simulink model "MIMO_FLOATING_POINT"  (R2023b)
settings: Solver=VariableStepAuto  StartTime=0.0  StopTime=1000  RelTol=1e-3
libraries: dspsigops x80, commchan3 x4, commdigbbndpm3 x2, commfilt2 x2, commsink2 x1, simulink x1, commrandsrc3 x1
(part 3 of 3)

== system MIMO_FLOATING_POINT/Transceiver5/Interpolation /E1(Z) ==
  Input1 : Inport
  10-12 : Gain  Gain=0.3078
  2-20 : Gain  Gain=0.0011
  4-18 : Gain  Gain=-0.0072
  6-16 : Gain  Gain=0.0263
  8-14 : Gain  Gain=-0.078
  Add{7..10,12..16} (9 alike) : Sum
  Delay{21,23,25,27,29,31,33,35,37} (9 alike) : Delay  DelayLength=1
  Output : Outport
  wires:
  8-14/1 -> Add13/1, Add9/1
  Delay29/1 -> Add12/2  "x[n-11]"
  Add14/1 -> Delay35/1
  Input1/1 -> 2-20/1, 4-18/1, 6-16/1, 8-14/1, 10-12/1
  Add8/1 -> Delay25/1
  4-18/1 -> Add15/1, Add7/1
  Delay33/1 -> Add14/2  "x[n-15]"
  Add12/1 -> Delay31/1
  10-12/1 -> Add10/1, Add12/1
  Add9/1 -> Delay27/1
  Add16/1 -> Output/1
  Delay37/1 -> Add16/2  "x[n-19]"
  6-16/1 -> Add14/1, Add8/1
  Delay25/1 -> Add9/2  "x[n-7]"
  Add7/1 -> Delay23/1
  Add15/1 -> Delay37/1
  Delay23/1 -> Add8/2  "x[n-5]"
  Delay27/1 -> Add10/2  "x[n-9]"
  Delay31/1 -> Add13/2  "x[n-13]"
  Delay35/1 -> Add15/2  "x[n-17]"
  Delay21/1 -> Add7/2  "x[n-3]"
  2-20/1 -> Delay21/1, Add16/1
  Add13/1 -> Delay33/1
  Add10/1 -> Delay29/1

== system MIMO_FLOATING_POINT/Transceiver5/Interpolation /E2 ==
  In1 : Inport
  Delay3 : Delay  DelayLength=1
  Delay4 : Delay  DelayLength=1
  Delay5 : Delay  DelayLength=1
  Gain : Gain  Gain=10
  Gain1 : Gain  Gain=246
  Sum : Sum
  Sum1 : Sum
  Sum2 : Sum
  Out1 : Outport
  wires:
  In1/1 -> Gain1/1, Gain/1
  Sum1/1 -> Delay5/1
  Sum/1 -> Delay4/1
  Gain1/1 -> Sum1/1, Sum/1
  Delay3/1 -> Sum/2
  Delay4/1 -> Sum1/2
  Gain/1 -> Sum2/1, Delay3/1
  Delay5/1 -> Sum2/2
  Sum2/1 -> Out1/1

== system MIMO_FLOATING_POINT/Transceiver5/Interpolation /E3 ==
  In1 : Inport
  Delay3 : Delay  DelayLength=1
  Delay4 : Delay  DelayLength=1
  Delay5 : Delay  DelayLength=1
  Gain : Gain  Gain=4
  Gain1 : Gain  Gain=204
  Gain2 : Gain  Gain=284
  Gain3 : Gain  Gain=20
  Sum : Sum
  Sum1 : Sum
  Sum2 : Sum
  Out1 : Outport
  wires:
  In1/1 -> Gain2/1, Gain3/1, Gain1/1, Gain/1
  Sum1/1 -> Delay5/1
  Sum/1 -> Delay4/1
  Gain1/1 -> Sum/1
  Delay3/1 -> Sum/2
  Delay4/1 -> Sum1/2
  Gain3/1 -> Sum2/1
  Delay5/1 -> Sum2/2
  Gain/1 -> Delay3/1
  Sum2/1 -> Out1/1
  Gain2/1 -> Sum1/1

== system MIMO_FLOATING_POINT/Transceiver5/Interpolation /E4 ==
  In1 : Inport
  Delay3 : Delay  DelayLength=1
  Delay4 : Delay  DelayLength=1
  Delay5 : Delay  DelayLength=1
  Gain : Gain
  Gain1 : Gain  Gain=161
  Gain2 : Gain  Gain=315
  Gain3 : Gain  Gain=35
  Sum : Sum
  Sum1 : Sum
  Sum2 : Sum
  Out1 : Outport
  wires:
  In1/1 -> Gain2/1, Gain3/1, Gain1/1, Gain/1
  Sum1/1 -> Delay5/1
  Sum/1 -> Delay4/1
  Gain1/1 -> Sum/1
  Delay3/1 -> Sum/2
  Delay4/1 -> Sum1/2
  Gain3/1 -> Sum2/1
  Delay5/1 -> Sum2/2
  Gain/1 -> Delay3/1
  Sum2/1 -> Out1/1
  Gain2/1 -> Sum1/1

== system MIMO_FLOATING_POINT/Transceiver5/Interpolation /E5 ==
  In1 : Inport
  Delay6 : Delay  DelayLength=1
  Delay7 : Delay  DelayLength=1
  Gain4 : Gain  Gain=120
  Gain5 : Gain  Gain=336
  Gain6 : Gain  Gain=56
  Sum4 : Sum
  Sum5 : Sum
  Out1 : Outport
  wires:
  Gain4/1 -> Delay6/1
  In1/1 -> Gain6/1, Gain5/1, Gain4/1
  Sum5/1 -> Out1/1
  Sum4/1 -> Delay7/1
  Delay7/1 -> Sum5/2
  Gain6/1 -> Sum5/1
  Gain5/1 -> Sum4/1
  Delay6/1 -> Sum4/2

== system MIMO_FLOATING_POINT/Transceiver5/Interpolation /E6 ==
  In1 : Inport
  Delay6 : Delay  DelayLength=1
  Delay7 : Delay  DelayLength=1
  Gain4 : Gain  Gain=84
  Gain5 : Gain  Gain=344
  Sum4 : Sum
  Sum5 : Sum
  Out1 : Outport
  wires:
  In1/1 -> Gain5/1, Gain4/1
  Sum5/1 -> Out1/1
  Sum4/1 -> Delay7/1
  Delay7/1 -> Sum5/2
  Gain4/1 -> Sum5/1, Delay6/1
  Gain5/1 -> Sum4/1
  Delay6/1 -> Sum4/2

== system MIMO_FLOATING_POINT/Transceiver5/Interpolation /E7 ==
  In1 : Inport
  Delay6 : Delay  DelayLength=1
  Delay7 : Delay  DelayLength=1
  Gain4 : Gain  Gain=56
  Gain5 : Gain  Gain=336
  Gain6 : Gain  Gain=120
  Sum4 : Sum
  Sum5 : Sum
  Out1 : Outport
  wires:
  Gain4/1 -> Delay6/1
  In1/1 -> Gain6/1, Gain5/1, Gain4/1
  Sum5/1 -> Out1/1
  Sum4/1 -> Delay7/1
  Delay7/1 -> Sum5/2
  Gain6/1 -> Sum5/1
  Gain5/1 -> Sum4/1
  Delay6/1 -> Sum4/2

== system MIMO_FLOATING_POINT/Transceiver5/Interpolation 1/E0 ==
  In1 : Inport
  Delay3 : Delay  DelayLength=1
  Delay4 : Delay  DelayLength=1
  Delay5 : Delay  DelayLength=1
  Gain : Gain  Gain=35
  Gain1 : Gain  Gain=315
  Gain2 : Gain  Gain=161
  Gain3 : Gain
  Sum : Sum
  Sum1 : Sum
  Sum2 : Sum
  Out1 : Outport
  wires:
  In1/1 -> Gain2/1, Gain3/1, Gain1/1, Gain/1
  Sum1/1 -> Delay5/1
  Sum/1 -> Delay4/1
  Gain1/1 -> Sum/1
  Delay3/1 -> Sum/2
  Delay4/1 -> Sum1/2
  Gain3/1 -> Sum2/1
  Delay5/1 -> Sum2/2
  Gain/1 -> Delay3/1
  Sum2/1 -> Out1/1
  Gain2/1 -> Sum1/1

== system MIMO_FLOATING_POINT/Transceiver5/Interpolation 1/E0(Z) ==
  Input : Inport
  Delay : Delay  DelayLength=5
  Gain : Gain  Gain=0.5
  Out1 : Outport
  wires:
  Input/1 -> Gain/1
  Delay/1 -> Out1/1
  Gain/1 -> Delay/1

== system MIMO_FLOATING_POINT/Transceiver5/Interpolation 1/E1 ==
  In1 : Inport
  Delay3 : Delay  DelayLength=1
  Delay4 : Delay  DelayLength=1
  Delay5 : Delay  DelayLength=1
  Gain : Gain  Gain=20
  Gain1 : Gain  Gain=284
  Gain2 : Gain  Gain=204
  Gain3 : Gain  Gain=4
  Sum : Sum
  Sum1 : Sum
  Sum2 : Sum
  Out1 : Outport
  wires:
  In1/1 -> Gain2/1, Gain3/1, Gain1/1, Gain/1
  Sum1/1 -> Delay5/1
  Sum/1 -> Delay4/1
  Gain1/1 -> Sum/1
  Delay3/1 -> Sum/2
  Delay4/1 -> Sum1/2
  Gain3/1 -> Sum2/1
  Delay5/1 -> Sum2/2
  Gain/1 -> Delay3/1
  Sum2/1 -> Out1/1
  Gain2/1 -> Sum1/1

== system MIMO_FLOATING_POINT/Transceiver5/Interpolation 1/E1(Z) ==
  Input1 : Inport
  10-12 : Gain  Gain=0.3078
  2-20 : Gain  Gain=0.0011
  4-18 : Gain  Gain=-0.0072
  6-16 : Gain  Gain=0.0263
  8-14 : Gain  Gain=-0.078
  Add{7..10,12..16} (9 alike) : Sum
  Delay{21,23,25,27,29,31,33,35,37} (9 alike) : Delay  DelayLength=1
  Output : Outport
  wires:
  8-14/1 -> Add13/1, Add9/1
  Delay29/1 -> Add12/2  "x[n-11]"
  Add14/1 -> Delay35/1
  Input1/1 -> 2-20/1, 4-18/1, 6-16/1, 8-14/1, 10-12/1
  Add8/1 -> Delay25/1
  4-18/1 -> Add15/1, Add7/1
  Delay33/1 -> Add14/2  "x[n-15]"
  Add12/1 -> Delay31/1
  10-12/1 -> Add10/1, Add12/1
  Add9/1 -> Delay27/1
  Add16/1 -> Output/1
  Delay37/1 -> Add16/2  "x[n-19]"
  6-16/1 -> Add14/1, Add8/1
  Delay25/1 -> Add9/2  "x[n-7]"
  Add7/1 -> Delay23/1
  Add15/1 -> Delay37/1
  Delay23/1 -> Add8/2  "x[n-5]"
  Delay27/1 -> Add10/2  "x[n-9]"
  Delay31/1 -> Add13/2  "x[n-13]"
  Delay35/1 -> Add15/2  "x[n-17]"
  Delay21/1 -> Add7/2  "x[n-3]"
  2-20/1 -> Delay21/1, Add16/1
  Add13/1 -> Delay33/1
  Add10/1 -> Delay29/1

== system MIMO_FLOATING_POINT/Transceiver5/Interpolation 1/E2 ==
  In1 : Inport
  Delay3 : Delay  DelayLength=1
  Delay4 : Delay  DelayLength=1
  Delay5 : Delay  DelayLength=1
  Gain : Gain  Gain=10
  Gain1 : Gain  Gain=246
  Sum : Sum
  Sum1 : Sum
  Sum2 : Sum
  Out1 : Outport
  wires:
  In1/1 -> Gain1/1, Gain/1
  Sum1/1 -> Delay5/1
  Sum/1 -> Delay4/1
  Gain1/1 -> Sum1/1, Sum/1
  Delay3/1 -> Sum/2
  Delay4/1 -> Sum1/2
  Gain/1 -> Sum2/1, Delay3/1
  Delay5/1 -> Sum2/2
  Sum2/1 -> Out1/1

== system MIMO_FLOATING_POINT/Transceiver5/Interpolation 1/E3 ==
  In1 : Inport
  Delay3 : Delay  DelayLength=1
  Delay4 : Delay  DelayLength=1
  Delay5 : Delay  DelayLength=1
  Gain : Gain  Gain=4
  Gain1 : Gain  Gain=204
  Gain2 : Gain  Gain=284
  Gain3 : Gain  Gain=20
  Sum : Sum
  Sum1 : Sum
  Sum2 : Sum
  Out1 : Outport
  wires:
  In1/1 -> Gain2/1, Gain3/1, Gain1/1, Gain/1
  Sum1/1 -> Delay5/1
  Sum/1 -> Delay4/1
  Gain1/1 -> Sum/1
  Delay3/1 -> Sum/2
  Delay4/1 -> Sum1/2
  Gain3/1 -> Sum2/1
  Delay5/1 -> Sum2/2
  Gain/1 -> Delay3/1
  Sum2/1 -> Out1/1
  Gain2/1 -> Sum1/1

== system MIMO_FLOATING_POINT/Transceiver5/Interpolation 1/E4 ==
  In1 : Inport
  Delay3 : Delay  DelayLength=1
  Delay4 : Delay  DelayLength=1
  Delay5 : Delay  DelayLength=1
  Gain : Gain
  Gain1 : Gain  Gain=161
  Gain2 : Gain  Gain=315
  Gain3 : Gain  Gain=35
  Sum : Sum
  Sum1 : Sum
  Sum2 : Sum
  Out1 : Outport
  wires:
  In1/1 -> Gain2/1, Gain3/1, Gain1/1, Gain/1
  Sum1/1 -> Delay5/1
  Sum/1 -> Delay4/1
  Gain1/1 -> Sum/1
  Delay3/1 -> Sum/2
  Delay4/1 -> Sum1/2
  Gain3/1 -> Sum2/1
  Delay5/1 -> Sum2/2
  Gain/1 -> Delay3/1
  Sum2/1 -> Out1/1
  Gain2/1 -> Sum1/1

== system MIMO_FLOATING_POINT/Transceiver5/Interpolation 1/E5 ==
  In1 : Inport
  Delay6 : Delay  DelayLength=1
  Delay7 : Delay  DelayLength=1
  Gain4 : Gain  Gain=120
  Gain5 : Gain  Gain=336
  Gain6 : Gain  Gain=56
  Sum4 : Sum
  Sum5 : Sum
  Out1 : Outport
  wires:
  Gain4/1 -> Delay6/1
  In1/1 -> Gain6/1, Gain5/1, Gain4/1
  Sum5/1 -> Out1/1
  Sum4/1 -> Delay7/1
  Delay7/1 -> Sum5/2
  Gain6/1 -> Sum5/1
  Gain5/1 -> Sum4/1
  Delay6/1 -> Sum4/2

== system MIMO_FLOATING_POINT/Transceiver5/Interpolation 1/E6 ==
  In1 : Inport
  Delay6 : Delay  DelayLength=1
  Delay7 : Delay  DelayLength=1
  Gain4 : Gain  Gain=84
  Gain5 : Gain  Gain=344
  Sum4 : Sum
  Sum5 : Sum
  Out1 : Outport
  wires:
  In1/1 -> Gain5/1, Gain4/1
  Sum5/1 -> Out1/1
  Sum4/1 -> Delay7/1
  Delay7/1 -> Sum5/2
  Gain4/1 -> Sum5/1, Delay6/1
  Gain5/1 -> Sum4/1
  Delay6/1 -> Sum4/2

== system MIMO_FLOATING_POINT/Transceiver5/Interpolation 1/E7 ==
  In1 : Inport
  Delay6 : Delay  DelayLength=1
  Delay7 : Delay  DelayLength=1
  Gain4 : Gain  Gain=56
  Gain5 : Gain  Gain=336
  Gain6 : Gain  Gain=120
  Sum4 : Sum
  Sum5 : Sum
  Out1 : Outport
  wires:
  Gain4/1 -> Delay6/1
  In1/1 -> Gain6/1, Gain5/1, Gain4/1
  Sum5/1 -> Out1/1
  Sum4/1 -> Delay7/1
  Delay7/1 -> Sum5/2
  Gain6/1 -> Sum5/1
  Gain5/1 -> Sum4/1
  Delay6/1 -> Sum4/2

== system MIMO_FLOATING_POINT/Transceiver6/ADC 1/SigmaDelta ADC ==
  note: c1
  In : Inport
  Discrete Transfer Fcn : DiscreteTransferFcn  Denominator=[1 -1]
  Discrete Transfer Fcn1 : DiscreteTransferFcn  Numerator=[1 0]  Denominator=[1 -1]
  Discrete Transfer Fcn2 : DiscreteTransferFcn  Denominator=[1 -1]
  Discrete Transfer Fcn3 : DiscreteTransferFcn  Numerator=[1 0]  Denominator=[1 -1]
  Discrete Transfer Fcn4 : DiscreteTransferFcn  Denominator=[1 -1]
  Discrete Transfer Fcn5 : DiscreteTransferFcn  Numerator=[1 0]  Denominator=[1 -1]
  Sign : Signum
  Sum : Sum  Inputs=-++  InputSameDT=on  SaturateOnIntegerOverflow=on  OutDataTypeStr=Inherit: Same as first input
  Sum1 : Sum  Inputs=-+  InputSameDT=on  SaturateOnIntegerOverflow=on  OutDataTypeStr=Inherit: Same as first input
  Sum3 : Sum  Inputs=-+  InputSameDT=on  SaturateOnIntegerOverflow=on  OutDataTypeStr=Inherit: Same as first input
  Sum4 : Sum  Inputs=++++++  InputSameDT=on  SaturateOnIntegerOverflow=on  OutDataTypeStr=Inherit: Same as first input
  a : Gain  Gain=-1  SaturateOnIntegerOverflow=on  OutDataTypeStr=Inherit: Same as input  ParamDataTypeStr=Inherit: Same as input
  a1 : Gain  Gain=0.556869897897495  SaturateOnIntegerOverflow=on  OutDataTypeStr=Inherit: Same as input  ParamDataTypeStr=Inherit: Same as input
  a2 : Gain  Gain=-0.556869897925717  SaturateOnIntegerOverflow=on  OutDataTypeStr=Inherit: Same as input  ParamDataTypeStr=Inherit: Same as input
  a3 : Gain  Gain=5.57074843011795e-10  SaturateOnIntegerOverflow=on  OutDataTypeStr=Inherit: Same as input  ParamDataTypeStr=Inherit: Same as input
  a4 : Gain  Gain=-0.239860502762260  SaturateOnIntegerOverflow=on  OutDataTypeStr=Inherit: Same as input  ParamDataTypeStr=Inherit: Same as input
  a5 : Gain  Gain=-0.0411685762497780  SaturateOnIntegerOverflow=on  OutDataTypeStr=Inherit: Same as input  ParamDataTypeStr=Inherit: Same as input
  a6 : Gain  Gain=0.0229325751731016  SaturateOnIntegerOverflow=on  OutDataTypeStr=Inherit: Same as input  ParamDataTypeStr=Inherit: Same as input
  gc1 : Gain  Gain=2.00000000000000  SaturateOnIntegerOverflow=on  OutDataTypeStr=Inherit: Same as input  ParamDataTypeStr=Inherit: Same as input
  gc2 : Gain  Gain=2.07602752770857  SaturateOnIntegerOverflow=on  OutDataTypeStr=Inherit: Same as input  ParamDataTypeStr=Inherit: Same as input
  gc3 : Gain  Gain=1.92397247229143  SaturateOnIntegerOverflow=on  OutDataTypeStr=Inherit: Same as input  ParamDataTypeStr=Inherit: Same as input
  Out : Outport
  wires:
  gc1/1 -> Sum/1
  a5/1 -> Sum4/2
  Discrete Transfer Fcn2/1 -> Discrete Transfer Fcn3/1, a3/1
  Sum4/1 -> Sign/1
  Sum1/1 -> Discrete Transfer Fcn2/1
  Sum/1 -> Discrete Transfer Fcn/1
  a1/1 -> Sum4/6
  gc2/1 -> Sum1/1
  a/1 -> Sum/3
  Discrete Transfer Fcn3/1 -> a4/1, Sum3/2, gc2/1
  Discrete Transfer Fcn5/1 -> a6/1, gc3/1
  Discrete Transfer Fcn1/1 -> a2/1, gc1/1, Sum1/2
  In/1 -> Sum/2
  Sign/1 -> Out/1, a/1
  gc3/1 -> Sum3/1
  a3/1 -> Sum4/4
  a4/1 -> Sum4/3
  a2/1 -> Sum4/5
  Discrete Transfer Fcn/1 -> Discrete Transfer Fcn1/1, a1/1
  Sum3/1 -> Discrete Transfer Fcn4/1
  Discrete Transfer Fcn4/1 -> Discrete Transfer Fcn5/1, a5/1
  a6/1 -> Sum4/1

== system MIMO_FLOATING_POINT/Transceiver6/Interpolation /E0 ==
  In1 : Inport
  Delay3 : Delay  DelayLength=1
  Delay4 : Delay  DelayLength=1
  Delay5 : Delay  DelayLength=1
  Gain : Gain  Gain=35
  Gain1 : Gain  Gain=315
  Gain2 : Gain  Gain=161
  Gain3 : Gain
  Sum : Sum
  Sum1 : Sum
  Sum2 : Sum
  Out1 : Outport
  wires:
  In1/1 -> Gain2/1, Gain3/1, Gain1/1, Gain/1
  Sum1/1 -> Delay5/1
  Sum/1 -> Delay4/1
  Gain1/1 -> Sum/1
  Delay3/1 -> Sum/2
  Delay4/1 -> Sum1/2
  Gain3/1 -> Sum2/1
  Delay5/1 -> Sum2/2
  Gain/1 -> Delay3/1
  Sum2/1 -> Out1/1
  Gain2/1 -> Sum1/1

== system MIMO_FLOATING_POINT/Transceiver6/Interpolation /E0(Z) ==
  Input : Inport
  Delay : Delay  DelayLength=5
  Gain : Gain  Gain=0.5
  Out1 : Outport
  wires:
  Input/1 -> Gain/1
  Delay/1 -> Out1/1
  Gain/1 -> Delay/1

== system MIMO_FLOATING_POINT/Transceiver6/Interpolation /E1 ==
  In1 : Inport
  Delay3 : Delay  DelayLength=1
  Delay4 : Delay  DelayLength=1
  Delay5 : Delay  DelayLength=1
  Gain : Gain  Gain=20
  Gain1 : Gain  Gain=284
  Gain2 : Gain  Gain=204
  Gain3 : Gain  Gain=4
  Sum : Sum
  Sum1 : Sum
  Sum2 : Sum
  Out1 : Outport
  wires:
  In1/1 -> Gain2/1, Gain3/1, Gain1/1, Gain/1
  Sum1/1 -> Delay5/1
  Sum/1 -> Delay4/1
  Gain1/1 -> Sum/1
  Delay3/1 -> Sum/2
  Delay4/1 -> Sum1/2
  Gain3/1 -> Sum2/1
  Delay5/1 -> Sum2/2
  Gain/1 -> Delay3/1
  Sum2/1 -> Out1/1
  Gain2/1 -> Sum1/1

== system MIMO_FLOATING_POINT/Transceiver6/Interpolation /E1(Z) ==
  Input1 : Inport
  10-12 : Gain  Gain=0.3078
  2-20 : Gain  Gain=0.0011
  4-18 : Gain  Gain=-0.0072
  6-16 : Gain  Gain=0.0263
  8-14 : Gain  Gain=-0.078
  Add{7..10,12..16} (9 alike) : Sum
  Delay{21,23,25,27,29,31,33,35,37} (9 alike) : Delay  DelayLength=1
  Output : Outport
  wires:
  8-14/1 -> Add13/1, Add9/1
  Delay29/1 -> Add12/2  "x[n-11]"
  Add14/1 -> Delay35/1
  Input1/1 -> 2-20/1, 4-18/1, 6-16/1, 8-14/1, 10-12/1
  Add8/1 -> Delay25/1
  4-18/1 -> Add15/1, Add7/1
  Delay33/1 -> Add14/2  "x[n-15]"
  Add12/1 -> Delay31/1
  10-12/1 -> Add10/1, Add12/1
  Add9/1 -> Delay27/1
  Add16/1 -> Output/1
  Delay37/1 -> Add16/2  "x[n-19]"
  6-16/1 -> Add14/1, Add8/1
  Delay25/1 -> Add9/2  "x[n-7]"
  Add7/1 -> Delay23/1
  Add15/1 -> Delay37/1
  Delay23/1 -> Add8/2  "x[n-5]"
  Delay27/1 -> Add10/2  "x[n-9]"
  Delay31/1 -> Add13/2  "x[n-13]"
  Delay35/1 -> Add15/2  "x[n-17]"
  Delay21/1 -> Add7/2  "x[n-3]"
  2-20/1 -> Delay21/1, Add16/1
  Add13/1 -> Delay33/1
  Add10/1 -> Delay29/1

== system MIMO_FLOATING_POINT/Transceiver6/Interpolation /E2 ==
  In1 : Inport
  Delay3 : Delay  DelayLength=1
  Delay4 : Delay  DelayLength=1
  Delay5 : Delay  DelayLength=1
  Gain : Gain  Gain=10
  Gain1 : Gain  Gain=246
  Sum : Sum
  Sum1 : Sum
  Sum2 : Sum
  Out1 : Outport
  wires:
  In1/1 -> Gain1/1, Gain/1
  Sum1/1 -> Delay5/1
  Sum/1 -> Delay4/1
  Gain1/1 -> Sum1/1, Sum/1
  Delay3/1 -> Sum/2
  Delay4/1 -> Sum1/2
  Gain/1 -> Sum2/1, Delay3/1
  Delay5/1 -> Sum2/2
  Sum2/1 -> Out1/1

== system MIMO_FLOATING_POINT/Transceiver6/Interpolation /E3 ==
  In1 : Inport
  Delay3 : Delay  DelayLength=1
  Delay4 : Delay  DelayLength=1
  Delay5 : Delay  DelayLength=1
  Gain : Gain  Gain=4
  Gain1 : Gain  Gain=204
  Gain2 : Gain  Gain=284
  Gain3 : Gain  Gain=20
  Sum : Sum
  Sum1 : Sum
  Sum2 : Sum
  Out1 : Outport
  wires:
  In1/1 -> Gain2/1, Gain3/1, Gain1/1, Gain/1
  Sum1/1 -> Delay5/1
  Sum/1 -> Delay4/1
  Gain1/1 -> Sum/1
  Delay3/1 -> Sum/2
  Delay4/1 -> Sum1/2
  Gain3/1 -> Sum2/1
  Delay5/1 -> Sum2/2
  Gain/1 -> Delay3/1
  Sum2/1 -> Out1/1
  Gain2/1 -> Sum1/1

== system MIMO_FLOATING_POINT/Transceiver6/Interpolation /E4 ==
  In1 : Inport
  Delay3 : Delay  DelayLength=1
  Delay4 : Delay  DelayLength=1
  Delay5 : Delay  DelayLength=1
  Gain : Gain
  Gain1 : Gain  Gain=161
  Gain2 : Gain  Gain=315
  Gain3 : Gain  Gain=35
  Sum : Sum
  Sum1 : Sum
  Sum2 : Sum
  Out1 : Outport
  wires:
  In1/1 -> Gain2/1, Gain3/1, Gain1/1, Gain/1
  Sum1/1 -> Delay5/1
  Sum/1 -> Delay4/1
  Gain1/1 -> Sum/1
  Delay3/1 -> Sum/2
  Delay4/1 -> Sum1/2
  Gain3/1 -> Sum2/1
  Delay5/1 -> Sum2/2
  Gain/1 -> Delay3/1
  Sum2/1 -> Out1/1
  Gain2/1 -> Sum1/1

== system MIMO_FLOATING_POINT/Transceiver6/Interpolation /E5 ==
  In1 : Inport
  Delay6 : Delay  DelayLength=1
  Delay7 : Delay  DelayLength=1
  Gain4 : Gain  Gain=120
  Gain5 : Gain  Gain=336
  Gain6 : Gain  Gain=56
  Sum4 : Sum
  Sum5 : Sum
  Out1 : Outport
  wires:
  Gain4/1 -> Delay6/1
  In1/1 -> Gain6/1, Gain5/1, Gain4/1
  Sum5/1 -> Out1/1
  Sum4/1 -> Delay7/1
  Delay7/1 -> Sum5/2
  Gain6/1 -> Sum5/1
  Gain5/1 -> Sum4/1
  Delay6/1 -> Sum4/2

== system MIMO_FLOATING_POINT/Transceiver6/Interpolation /E6 ==
  In1 : Inport
  Delay6 : Delay  DelayLength=1
  Delay7 : Delay  DelayLength=1
  Gain4 : Gain  Gain=84
  Gain5 : Gain  Gain=344
  Sum4 : Sum
  Sum5 : Sum
  Out1 : Outport
  wires:
  In1/1 -> Gain5/1, Gain4/1
  Sum5/1 -> Out1/1
  Sum4/1 -> Delay7/1
  Delay7/1 -> Sum5/2
  Gain4/1 -> Sum5/1, Delay6/1
  Gain5/1 -> Sum4/1
  Delay6/1 -> Sum4/2

== system MIMO_FLOATING_POINT/Transceiver6/Interpolation /E7 ==
  In1 : Inport
  Delay6 : Delay  DelayLength=1
  Delay7 : Delay  DelayLength=1
  Gain4 : Gain  Gain=56
  Gain5 : Gain  Gain=336
  Gain6 : Gain  Gain=120
  Sum4 : Sum
  Sum5 : Sum
  Out1 : Outport
  wires:
  Gain4/1 -> Delay6/1
  In1/1 -> Gain6/1, Gain5/1, Gain4/1
  Sum5/1 -> Out1/1
  Sum4/1 -> Delay7/1
  Delay7/1 -> Sum5/2
  Gain6/1 -> Sum5/1
  Gain5/1 -> Sum4/1
  Delay6/1 -> Sum4/2

== system MIMO_FLOATING_POINT/Transceiver6/Interpolation 1/E0 ==
  In1 : Inport
  Delay3 : Delay  DelayLength=1
  Delay4 : Delay  DelayLength=1
  Delay5 : Delay  DelayLength=1
  Gain : Gain  Gain=35
  Gain1 : Gain  Gain=315
  Gain2 : Gain  Gain=161
  Gain3 : Gain
  Sum : Sum
  Sum1 : Sum
  Sum2 : Sum
  Out1 : Outport
  wires:
  In1/1 -> Gain2/1, Gain3/1, Gain1/1, Gain/1
  Sum1/1 -> Delay5/1
  Sum/1 -> Delay4/1
  Gain1/1 -> Sum/1
  Delay3/1 -> Sum/2
  Delay4/1 -> Sum1/2
  Gain3/1 -> Sum2/1
  Delay5/1 -> Sum2/2
  Gain/1 -> Delay3/1
  Sum2/1 -> Out1/1
  Gain2/1 -> Sum1/1

== system MIMO_FLOATING_POINT/Transceiver6/Interpolation 1/E0(Z) ==
  Input : Inport
  Delay : Delay  DelayLength=5
  Gain : Gain  Gain=0.5
  Out1 : Outport
  wires:
  Input/1 -> Gain/1
  Delay/1 -> Out1/1
  Gain/1 -> Delay/1

== system MIMO_FLOATING_POINT/Transceiver6/Interpolation 1/E1 ==
  In1 : Inport
  Delay3 : Delay  DelayLength=1
  Delay4 : Delay  DelayLength=1
  Delay5 : Delay  DelayLength=1
  Gain : Gain  Gain=20
  Gain1 : Gain  Gain=284
  Gain2 : Gain  Gain=204
  Gain3 : Gain  Gain=4
  Sum : Sum
  Sum1 : Sum
  Sum2 : Sum
  Out1 : Outport
  wires:
  In1/1 -> Gain2/1, Gain3/1, Gain1/1, Gain/1
  Sum1/1 -> Delay5/1
  Sum/1 -> Delay4/1
  Gain1/1 -> Sum/1
  Delay3/1 -> Sum/2
  Delay4/1 -> Sum1/2
  Gain3/1 -> Sum2/1
  Delay5/1 -> Sum2/2
  Gain/1 -> Delay3/1
  Sum2/1 -> Out1/1
  Gain2/1 -> Sum1/1

== system MIMO_FLOATING_POINT/Transceiver6/Interpolation 1/E1(Z) ==
  Input1 : Inport
  10-12 : Gain  Gain=0.3078
  2-20 : Gain  Gain=0.0011
  4-18 : Gain  Gain=-0.0072
  6-16 : Gain  Gain=0.0263
  8-14 : Gain  Gain=-0.078
  Add{7..10,12..16} (9 alike) : Sum
  Delay{21,23,25,27,29,31,33,35,37} (9 alike) : Delay  DelayLength=1
  Output : Outport
  wires:
  8-14/1 -> Add13/1, Add9/1
  Delay29/1 -> Add12/2  "x[n-11]"
  Add14/1 -> Delay35/1
  Input1/1 -> 2-20/1, 4-18/1, 6-16/1, 8-14/1, 10-12/1
  Add8/1 -> Delay25/1
  4-18/1 -> Add15/1, Add7/1
  Delay33/1 -> Add14/2  "x[n-15]"
  Add12/1 -> Delay31/1
  10-12/1 -> Add10/1, Add12/1
  Add9/1 -> Delay27/1
  Add16/1 -> Output/1
  Delay37/1 -> Add16/2  "x[n-19]"
  6-16/1 -> Add14/1, Add8/1
  Delay25/1 -> Add9/2  "x[n-7]"
  Add7/1 -> Delay23/1
  Add15/1 -> Delay37/1
  Delay23/1 -> Add8/2  "x[n-5]"
  Delay27/1 -> Add10/2  "x[n-9]"
  Delay31/1 -> Add13/2  "x[n-13]"
  Delay35/1 -> Add15/2  "x[n-17]"
  Delay21/1 -> Add7/2  "x[n-3]"
  2-20/1 -> Delay21/1, Add16/1
  Add13/1 -> Delay33/1
  Add10/1 -> Delay29/1

== system MIMO_FLOATING_POINT/Transceiver6/Interpolation 1/E2 ==
  In1 : Inport
  Delay3 : Delay  DelayLength=1
  Delay4 : Delay  DelayLength=1
  Delay5 : Delay  DelayLength=1
  Gain : Gain  Gain=10
  Gain1 : Gain  Gain=246
  Sum : Sum
  Sum1 : Sum
  Sum2 : Sum
  Out1 : Outport
  wires:
  In1/1 -> Gain1/1, Gain/1
  Sum1/1 -> Delay5/1
  Sum/1 -> Delay4/1
  Gain1/1 -> Sum1/1, Sum/1
  Delay3/1 -> Sum/2
  Delay4/1 -> Sum1/2
  Gain/1 -> Sum2/1, Delay3/1
  Delay5/1 -> Sum2/2
  Sum2/1 -> Out1/1

== system MIMO_FLOATING_POINT/Transceiver6/Interpolation 1/E3 ==
  In1 : Inport
  Delay3 : Delay  DelayLength=1
  Delay4 : Delay  DelayLength=1
  Delay5 : Delay  DelayLength=1
  Gain : Gain  Gain=4
  Gain1 : Gain  Gain=204
  Gain2 : Gain  Gain=284
  Gain3 : Gain  Gain=20
  Sum : Sum
  Sum1 : Sum
  Sum2 : Sum
  Out1 : Outport
  wires:
  In1/1 -> Gain2/1, Gain3/1, Gain1/1, Gain/1
  Sum1/1 -> Delay5/1
  Sum/1 -> Delay4/1
  Gain1/1 -> Sum/1
  Delay3/1 -> Sum/2
  Delay4/1 -> Sum1/2
  Gain3/1 -> Sum2/1
  Delay5/1 -> Sum2/2
  Gain/1 -> Delay3/1
  Sum2/1 -> Out1/1
  Gain2/1 -> Sum1/1

== system MIMO_FLOATING_POINT/Transceiver6/Interpolation 1/E4 ==
  In1 : Inport
  Delay3 : Delay  DelayLength=1
  Delay4 : Delay  DelayLength=1
  Delay5 : Delay  DelayLength=1
  Gain : Gain
  Gain1 : Gain  Gain=161
  Gain2 : Gain  Gain=315
  Gain3 : Gain  Gain=35
  Sum : Sum
  Sum1 : Sum
  Sum2 : Sum
  Out1 : Outport
  wires:
  In1/1 -> Gain2/1, Gain3/1, Gain1/1, Gain/1
  Sum1/1 -> Delay5/1
  Sum/1 -> Delay4/1
  Gain1/1 -> Sum/1
  Delay3/1 -> Sum/2
  Delay4/1 -> Sum1/2
  Gain3/1 -> Sum2/1
  Delay5/1 -> Sum2/2
  Gain/1 -> Delay3/1
  Sum2/1 -> Out1/1
  Gain2/1 -> Sum1/1

== system MIMO_FLOATING_POINT/Transceiver6/Interpolation 1/E5 ==
  In1 : Inport
  Delay6 : Delay  DelayLength=1
  Delay7 : Delay  DelayLength=1
  Gain4 : Gain  Gain=120
  Gain5 : Gain  Gain=336
  Gain6 : Gain  Gain=56
  Sum4 : Sum
  Sum5 : Sum
  Out1 : Outport
  wires:
  Gain4/1 -> Delay6/1
  In1/1 -> Gain6/1, Gain5/1, Gain4/1
  Sum5/1 -> Out1/1
  Sum4/1 -> Delay7/1
  Delay7/1 -> Sum5/2
  Gain6/1 -> Sum5/1
  Gain5/1 -> Sum4/1
  Delay6/1 -> Sum4/2

== system MIMO_FLOATING_POINT/Transceiver6/Interpolation 1/E6 ==
  In1 : Inport
  Delay6 : Delay  DelayLength=1
  Delay7 : Delay  DelayLength=1
  Gain4 : Gain  Gain=84
  Gain5 : Gain  Gain=344
  Sum4 : Sum
  Sum5 : Sum
  Out1 : Outport
  wires:
  In1/1 -> Gain5/1, Gain4/1
  Sum5/1 -> Out1/1
  Sum4/1 -> Delay7/1
  Delay7/1 -> Sum5/2
  Gain4/1 -> Sum5/1, Delay6/1
  Gain5/1 -> Sum4/1
  Delay6/1 -> Sum4/2

== system MIMO_FLOATING_POINT/Transceiver6/Interpolation 1/E7 ==
  In1 : Inport
  Delay6 : Delay  DelayLength=1
  Delay7 : Delay  DelayLength=1
  Gain4 : Gain  Gain=56
  Gain5 : Gain  Gain=336
  Gain6 : Gain  Gain=120
  Sum4 : Sum
  Sum5 : Sum
  Out1 : Outport
  wires:
  Gain4/1 -> Delay6/1
  In1/1 -> Gain6/1, Gain5/1, Gain4/1
  Sum5/1 -> Out1/1
  Sum4/1 -> Delay7/1
  Delay7/1 -> Sum5/2
  Gain6/1 -> Sum5/1
  Gain5/1 -> Sum4/1
  Delay6/1 -> Sum4/2

== system MIMO_FLOATING_POINT/Transceiver7/ADC 1/SigmaDelta ADC ==
  note: c1
  In : Inport
  Discrete Transfer Fcn : DiscreteTransferFcn  Denominator=[1 -1]
  Discrete Transfer Fcn1 : DiscreteTransferFcn  Numerator=[1 0]  Denominator=[1 -1]
  Discrete Transfer Fcn2 : DiscreteTransferFcn  Denominator=[1 -1]
  Discrete Transfer Fcn3 : DiscreteTransferFcn  Numerator=[1 0]  Denominator=[1 -1]
  Discrete Transfer Fcn4 : DiscreteTransferFcn  Denominator=[1 -1]
  Discrete Transfer Fcn5 : DiscreteTransferFcn  Numerator=[1 0]  Denominator=[1 -1]
  Sign : Signum
  Sum : Sum  Inputs=-++  InputSameDT=on  SaturateOnIntegerOverflow=on  OutDataTypeStr=Inherit: Same as first input
  Sum1 : Sum  Inputs=-+  InputSameDT=on  SaturateOnIntegerOverflow=on  OutDataTypeStr=Inherit: Same as first input
  Sum3 : Sum  Inputs=-+  InputSameDT=on  SaturateOnIntegerOverflow=on  OutDataTypeStr=Inherit: Same as first input
  Sum4 : Sum  Inputs=++++++  InputSameDT=on  SaturateOnIntegerOverflow=on  OutDataTypeStr=Inherit: Same as first input
  a : Gain  Gain=-1  SaturateOnIntegerOverflow=on  OutDataTypeStr=Inherit: Same as input  ParamDataTypeStr=Inherit: Same as input
  a1 : Gain  Gain=0.556869897897495  SaturateOnIntegerOverflow=on  OutDataTypeStr=Inherit: Same as input  ParamDataTypeStr=Inherit: Same as input
  a2 : Gain  Gain=-0.556869897925717  SaturateOnIntegerOverflow=on  OutDataTypeStr=Inherit: Same as input  ParamDataTypeStr=Inherit: Same as input
  a3 : Gain  Gain=5.57074843011795e-10  SaturateOnIntegerOverflow=on  OutDataTypeStr=Inherit: Same as input  ParamDataTypeStr=Inherit: Same as input
  a4 : Gain  Gain=-0.239860502762260  SaturateOnIntegerOverflow=on  OutDataTypeStr=Inherit: Same as input  ParamDataTypeStr=Inherit: Same as input
  a5 : Gain  Gain=-0.0411685762497780  SaturateOnIntegerOverflow=on  OutDataTypeStr=Inherit: Same as input  ParamDataTypeStr=Inherit: Same as input
  a6 : Gain  Gain=0.0229325751731016  SaturateOnIntegerOverflow=on  OutDataTypeStr=Inherit: Same as input  ParamDataTypeStr=Inherit: Same as input
  gc1 : Gain  Gain=2.00000000000000  SaturateOnIntegerOverflow=on  OutDataTypeStr=Inherit: Same as input  ParamDataTypeStr=Inherit: Same as input
  gc2 : Gain  Gain=2.07602752770857  SaturateOnIntegerOverflow=on  OutDataTypeStr=Inherit: Same as input  ParamDataTypeStr=Inherit: Same as input
  gc3 : Gain  Gain=1.92397247229143  SaturateOnIntegerOverflow=on  OutDataTypeStr=Inherit: Same as input  ParamDataTypeStr=Inherit: Same as input
  Out : Outport
  wires:
  gc1/1 -> Sum/1
  a5/1 -> Sum4/2
  Discrete Transfer Fcn2/1 -> Discrete Transfer Fcn3/1, a3/1
  Sum4/1 -> Sign/1
  Sum1/1 -> Discrete Transfer Fcn2/1
  Sum/1 -> Discrete Transfer Fcn/1
  a1/1 -> Sum4/6
  gc2/1 -> Sum1/1
  a/1 -> Sum/3
  Discrete Transfer Fcn3/1 -> a4/1, Sum3/2, gc2/1
  Discrete Transfer Fcn5/1 -> a6/1, gc3/1
  Discrete Transfer Fcn1/1 -> a2/1, gc1/1, Sum1/2
  In/1 -> Sum/2
  Sign/1 -> Out/1, a/1
  gc3/1 -> Sum3/1
  a3/1 -> Sum4/4
  a4/1 -> Sum4/3
  a2/1 -> Sum4/5
  Discrete Transfer Fcn/1 -> Discrete Transfer Fcn1/1, a1/1
  Sum3/1 -> Discrete Transfer Fcn4/1
  Discrete Transfer Fcn4/1 -> Discrete Transfer Fcn5/1, a5/1
  a6/1 -> Sum4/1

== system MIMO_FLOATING_POINT/Transceiver7/Interpolation /E0 ==
  In1 : Inport
  Delay3 : Delay  DelayLength=1
  Delay4 : Delay  DelayLength=1
  Delay5 : Delay  DelayLength=1
  Gain : Gain  Gain=35
  Gain1 : Gain  Gain=315
  Gain2 : Gain  Gain=161
  Gain3 : Gain
  Sum : Sum
  Sum1 : Sum
  Sum2 : Sum
  Out1 : Outport
  wires:
  In1/1 -> Gain2/1, Gain3/1, Gain1/1, Gain/1
  Sum1/1 -> Delay5/1
  Sum/1 -> Delay4/1
  Gain1/1 -> Sum/1
  Delay3/1 -> Sum/2
  Delay4/1 -> Sum1/2
  Gain3/1 -> Sum2/1
  Delay5/1 -> Sum2/2
  Gain/1 -> Delay3/1
  Sum2/1 -> Out1/1
  Gain2/1 -> Sum1/1

== system MIMO_FLOATING_POINT/Transceiver7/Interpolation /E0(Z) ==
  Input : Inport
  Delay : Delay  DelayLength=5
  Gain : Gain  Gain=0.5
  Out1 : Outport
  wires:
  Input/1 -> Gain/1
  Delay/1 -> Out1/1
  Gain/1 -> Delay/1

== system MIMO_FLOATING_POINT/Transceiver7/Interpolation /E1 ==
  In1 : Inport
  Delay3 : Delay  DelayLength=1
  Delay4 : Delay  DelayLength=1
  Delay5 : Delay  DelayLength=1
  Gain : Gain  Gain=20
  Gain1 : Gain  Gain=284
  Gain2 : Gain  Gain=204
  Gain3 : Gain  Gain=4
  Sum : Sum
  Sum1 : Sum
  Sum2 : Sum
  Out1 : Outport
  wires:
  In1/1 -> Gain2/1, Gain3/1, Gain1/1, Gain/1
  Sum1/1 -> Delay5/1
  Sum/1 -> Delay4/1
  Gain1/1 -> Sum/1
  Delay3/1 -> Sum/2
  Delay4/1 -> Sum1/2
  Gain3/1 -> Sum2/1
  Delay5/1 -> Sum2/2
  Gain/1 -> Delay3/1
  Sum2/1 -> Out1/1
  Gain2/1 -> Sum1/1

== system MIMO_FLOATING_POINT/Transceiver7/Interpolation /E1(Z) ==
  Input1 : Inport
  10-12 : Gain  Gain=0.3078
  2-20 : Gain  Gain=0.0011
  4-18 : Gain  Gain=-0.0072
  6-16 : Gain  Gain=0.0263
  8-14 : Gain  Gain=-0.078
  Add{7..10,12..16} (9 alike) : Sum
  Delay{21,23,25,27,29,31,33,35,37} (9 alike) : Delay  DelayLength=1
  Output : Outport
  wires:
  8-14/1 -> Add13/1, Add9/1
  Delay29/1 -> Add12/2  "x[n-11]"
  Add14/1 -> Delay35/1
  Input1/1 -> 2-20/1, 4-18/1, 6-16/1, 8-14/1, 10-12/1
  Add8/1 -> Delay25/1
  4-18/1 -> Add15/1, Add7/1
  Delay33/1 -> Add14/2  "x[n-15]"
  Add12/1 -> Delay31/1
  10-12/1 -> Add10/1, Add12/1
  Add9/1 -> Delay27/1
  Add16/1 -> Output/1
  Delay37/1 -> Add16/2  "x[n-19]"
  6-16/1 -> Add14/1, Add8/1
  Delay25/1 -> Add9/2  "x[n-7]"
  Add7/1 -> Delay23/1
  Add15/1 -> Delay37/1
  Delay23/1 -> Add8/2  "x[n-5]"
  Delay27/1 -> Add10/2  "x[n-9]"
  Delay31/1 -> Add13/2  "x[n-13]"
  Delay35/1 -> Add15/2  "x[n-17]"
  Delay21/1 -> Add7/2  "x[n-3]"
  2-20/1 -> Delay21/1, Add16/1
  Add13/1 -> Delay33/1
  Add10/1 -> Delay29/1

== system MIMO_FLOATING_POINT/Transceiver7/Interpolation /E2 ==
  In1 : Inport
  Delay3 : Delay  DelayLength=1
  Delay4 : Delay  DelayLength=1
  Delay5 : Delay  DelayLength=1
  Gain : Gain  Gain=10
  Gain1 : Gain  Gain=246
  Sum : Sum
  Sum1 : Sum
  Sum2 : Sum
  Out1 : Outport
  wires:
  In1/1 -> Gain1/1, Gain/1
  Sum1/1 -> Delay5/1
  Sum/1 -> Delay4/1
  Gain1/1 -> Sum1/1, Sum/1
  Delay3/1 -> Sum/2
  Delay4/1 -> Sum1/2
  Gain/1 -> Sum2/1, Delay3/1
  Delay5/1 -> Sum2/2
  Sum2/1 -> Out1/1

== system MIMO_FLOATING_POINT/Transceiver7/Interpolation /E3 ==
  In1 : Inport
  Delay3 : Delay  DelayLength=1
  Delay4 : Delay  DelayLength=1
  Delay5 : Delay  DelayLength=1
  Gain : Gain  Gain=4
  Gain1 : Gain  Gain=204
  Gain2 : Gain  Gain=284
  Gain3 : Gain  Gain=20
  Sum : Sum
  Sum1 : Sum
  Sum2 : Sum
  Out1 : Outport
  wires:
  In1/1 -> Gain2/1, Gain3/1, Gain1/1, Gain/1
  Sum1/1 -> Delay5/1
  Sum/1 -> Delay4/1
  Gain1/1 -> Sum/1
  Delay3/1 -> Sum/2
  Delay4/1 -> Sum1/2
  Gain3/1 -> Sum2/1
  Delay5/1 -> Sum2/2
  Gain/1 -> Delay3/1
  Sum2/1 -> Out1/1
  Gain2/1 -> Sum1/1

== system MIMO_FLOATING_POINT/Transceiver7/Interpolation /E4 ==
  In1 : Inport
  Delay3 : Delay  DelayLength=1
  Delay4 : Delay  DelayLength=1
  Delay5 : Delay  DelayLength=1
  Gain : Gain
  Gain1 : Gain  Gain=161
  Gain2 : Gain  Gain=315
  Gain3 : Gain  Gain=35
  Sum : Sum
  Sum1 : Sum
  Sum2 : Sum
  Out1 : Outport
  wires:
  In1/1 -> Gain2/1, Gain3/1, Gain1/1, Gain/1
  Sum1/1 -> Delay5/1
  Sum/1 -> Delay4/1
  Gain1/1 -> Sum/1
  Delay3/1 -> Sum/2
  Delay4/1 -> Sum1/2
  Gain3/1 -> Sum2/1
  Delay5/1 -> Sum2/2
  Gain/1 -> Delay3/1
  Sum2/1 -> Out1/1
  Gain2/1 -> Sum1/1

== system MIMO_FLOATING_POINT/Transceiver7/Interpolation /E5 ==
  In1 : Inport
  Delay6 : Delay  DelayLength=1
  Delay7 : Delay  DelayLength=1
  Gain4 : Gain  Gain=120
  Gain5 : Gain  Gain=336
  Gain6 : Gain  Gain=56
  Sum4 : Sum
  Sum5 : Sum
  Out1 : Outport
  wires:
  Gain4/1 -> Delay6/1
  In1/1 -> Gain6/1, Gain5/1, Gain4/1
  Sum5/1 -> Out1/1
  Sum4/1 -> Delay7/1
  Delay7/1 -> Sum5/2
  Gain6/1 -> Sum5/1
  Gain5/1 -> Sum4/1
  Delay6/1 -> Sum4/2

== system MIMO_FLOATING_POINT/Transceiver7/Interpolation /E6 ==
  In1 : Inport
  Delay6 : Delay  DelayLength=1
  Delay7 : Delay  DelayLength=1
  Gain4 : Gain  Gain=84
  Gain5 : Gain  Gain=344
  Sum4 : Sum
  Sum5 : Sum
  Out1 : Outport
  wires:
  In1/1 -> Gain5/1, Gain4/1
  Sum5/1 -> Out1/1
  Sum4/1 -> Delay7/1
  Delay7/1 -> Sum5/2
  Gain4/1 -> Sum5/1, Delay6/1
  Gain5/1 -> Sum4/1
  Delay6/1 -> Sum4/2

== system MIMO_FLOATING_POINT/Transceiver7/Interpolation /E7 ==
  In1 : Inport
  Delay6 : Delay  DelayLength=1
  Delay7 : Delay  DelayLength=1
  Gain4 : Gain  Gain=56
  Gain5 : Gain  Gain=336
  Gain6 : Gain  Gain=120
  Sum4 : Sum
  Sum5 : Sum
  Out1 : Outport
  wires:
  Gain4/1 -> Delay6/1
  In1/1 -> Gain6/1, Gain5/1, Gain4/1
  Sum5/1 -> Out1/1
  Sum4/1 -> Delay7/1
  Delay7/1 -> Sum5/2
  Gain6/1 -> Sum5/1
  Gain5/1 -> Sum4/1
  Delay6/1 -> Sum4/2

== system MIMO_FLOATING_POINT/Transceiver7/Interpolation 1/E0 ==
  In1 : Inport
  Delay3 : Delay  DelayLength=1
  Delay4 : Delay  DelayLength=1
  Delay5 : Delay  DelayLength=1
  Gain : Gain  Gain=35
  Gain1 : Gain  Gain=315
  Gain2 : Gain  Gain=161
  Gain3 : Gain
  Sum : Sum
  Sum1 : Sum
  Sum2 : Sum
  Out1 : Outport
  wires:
  In1/1 -> Gain2/1, Gain3/1, Gain1/1, Gain/1
  Sum1/1 -> Delay5/1
  Sum/1 -> Delay4/1
  Gain1/1 -> Sum/1
  Delay3/1 -> Sum/2
  Delay4/1 -> Sum1/2
  Gain3/1 -> Sum2/1
  Delay5/1 -> Sum2/2
  Gain/1 -> Delay3/1
  Sum2/1 -> Out1/1
  Gain2/1 -> Sum1/1

== system MIMO_FLOATING_POINT/Transceiver7/Interpolation 1/E0(Z) ==
  Input : Inport
  Delay : Delay  DelayLength=5
  Gain : Gain  Gain=0.5
  Out1 : Outport
  wires:
  Input/1 -> Gain/1
  Delay/1 -> Out1/1
  Gain/1 -> Delay/1

== system MIMO_FLOATING_POINT/Transceiver7/Interpolation 1/E1 ==
  In1 : Inport
  Delay3 : Delay  DelayLength=1
  Delay4 : Delay  DelayLength=1
  Delay5 : Delay  DelayLength=1
  Gain : Gain  Gain=20
  Gain1 : Gain  Gain=284
  Gain2 : Gain  Gain=204
  Gain3 : Gain  Gain=4
  Sum : Sum
  Sum1 : Sum
  Sum2 : Sum
  Out1 : Outport
  wires:
  In1/1 -> Gain2/1, Gain3/1, Gain1/1, Gain/1
  Sum1/1 -> Delay5/1
  Sum/1 -> Delay4/1
  Gain1/1 -> Sum/1
  Delay3/1 -> Sum/2
  Delay4/1 -> Sum1/2
  Gain3/1 -> Sum2/1
  Delay5/1 -> Sum2/2
  Gain/1 -> Delay3/1
  Sum2/1 -> Out1/1
  Gain2/1 -> Sum1/1

== system MIMO_FLOATING_POINT/Transceiver7/Interpolation 1/E1(Z) ==
  Input1 : Inport
  10-12 : Gain  Gain=0.3078
  2-20 : Gain  Gain=0.0011
  4-18 : Gain  Gain=-0.0072
  6-16 : Gain  Gain=0.0263
  8-14 : Gain  Gain=-0.078
  Add{7..10,12..16} (9 alike) : Sum
  Delay{21,23,25,27,29,31,33,35,37} (9 alike) : Delay  DelayLength=1
  Output : Outport
  wires:
  8-14/1 -> Add13/1, Add9/1
  Delay29/1 -> Add12/2  "x[n-11]"
  Add14/1 -> Delay35/1
  Input1/1 -> 2-20/1, 4-18/1, 6-16/1, 8-14/1, 10-12/1
  Add8/1 -> Delay25/1
  4-18/1 -> Add15/1, Add7/1
  Delay33/1 -> Add14/2  "x[n-15]"
  Add12/1 -> Delay31/1
  10-12/1 -> Add10/1, Add12/1
  Add9/1 -> Delay27/1
  Add16/1 -> Output/1
  Delay37/1 -> Add16/2  "x[n-19]"
  6-16/1 -> Add14/1, Add8/1
  Delay25/1 -> Add9/2  "x[n-7]"
  Add7/1 -> Delay23/1
  Add15/1 -> Delay37/1
  Delay23/1 -> Add8/2  "x[n-5]"
  Delay27/1 -> Add10/2  "x[n-9]"
  Delay31/1 -> Add13/2  "x[n-13]"
  Delay35/1 -> Add15/2  "x[n-17]"
  Delay21/1 -> Add7/2  "x[n-3]"
  2-20/1 -> Delay21/1, Add16/1
  Add13/1 -> Delay33/1
  Add10/1 -> Delay29/1

== system MIMO_FLOATING_POINT/Transceiver7/Interpolation 1/E2 ==
  In1 : Inport
  Delay3 : Delay  DelayLength=1
  Delay4 : Delay  DelayLength=1
  Delay5 : Delay  DelayLength=1
  Gain : Gain  Gain=10
  Gain1 : Gain  Gain=246
  Sum : Sum
  Sum1 : Sum
  Sum2 : Sum
  Out1 : Outport
  wires:
  In1/1 -> Gain1/1, Gain/1
  Sum1/1 -> Delay5/1
  Sum/1 -> Delay4/1
  Gain1/1 -> Sum1/1, Sum/1
  Delay3/1 -> Sum/2
  Delay4/1 -> Sum1/2
  Gain/1 -> Sum2/1, Delay3/1
  Delay5/1 -> Sum2/2
  Sum2/1 -> Out1/1

== system MIMO_FLOATING_POINT/Transceiver7/Interpolation 1/E3 ==
  In1 : Inport
  Delay3 : Delay  DelayLength=1
  Delay4 : Delay  DelayLength=1
  Delay5 : Delay  DelayLength=1
  Gain : Gain  Gain=4
  Gain1 : Gain  Gain=204
  Gain2 : Gain  Gain=284
  Gain3 : Gain  Gain=20
  Sum : Sum
  Sum1 : Sum
  Sum2 : Sum
  Out1 : Outport
  wires:
  In1/1 -> Gain2/1, Gain3/1, Gain1/1, Gain/1
  Sum1/1 -> Delay5/1
  Sum/1 -> Delay4/1
  Gain1/1 -> Sum/1
  Delay3/1 -> Sum/2
  Delay4/1 -> Sum1/2
  Gain3/1 -> Sum2/1
  Delay5/1 -> Sum2/2
  Gain/1 -> Delay3/1
  Sum2/1 -> Out1/1
  Gain2/1 -> Sum1/1

== system MIMO_FLOATING_POINT/Transceiver7/Interpolation 1/E4 ==
  In1 : Inport
  Delay3 : Delay  DelayLength=1
  Delay4 : Delay  DelayLength=1
  Delay5 : Delay  DelayLength=1
  Gain : Gain
  Gain1 : Gain  Gain=161
  Gain2 : Gain  Gain=315
  Gain3 : Gain  Gain=35
  Sum : Sum
  Sum1 : Sum
  Sum2 : Sum
  Out1 : Outport
  wires:
  In1/1 -> Gain2/1, Gain3/1, Gain1/1, Gain/1
  Sum1/1 -> Delay5/1
  Sum/1 -> Delay4/1
  Gain1/1 -> Sum/1
  Delay3/1 -> Sum/2
  Delay4/1 -> Sum1/2
  Gain3/1 -> Sum2/1
  Delay5/1 -> Sum2/2
  Gain/1 -> Delay3/1
  Sum2/1 -> Out1/1
  Gain2/1 -> Sum1/1

== system MIMO_FLOATING_POINT/Transceiver7/Interpolation 1/E5 ==
  In1 : Inport
  Delay6 : Delay  DelayLength=1
  Delay7 : Delay  DelayLength=1
  Gain4 : Gain  Gain=120
  Gain5 : Gain  Gain=336
  Gain6 : Gain  Gain=56
  Sum4 : Sum
  Sum5 : Sum
  Out1 : Outport
  wires:
  Gain4/1 -> Delay6/1
  In1/1 -> Gain6/1, Gain5/1, Gain4/1
  Sum5/1 -> Out1/1
  Sum4/1 -> Delay7/1
  Delay7/1 -> Sum5/2
  Gain6/1 -> Sum5/1
  Gain5/1 -> Sum4/1
  Delay6/1 -> Sum4/2

== system MIMO_FLOATING_POINT/Transceiver7/Interpolation 1/E6 ==
  In1 : Inport
  Delay6 : Delay  DelayLength=1
  Delay7 : Delay  DelayLength=1
  Gain4 : Gain  Gain=84
  Gain5 : Gain  Gain=344
  Sum4 : Sum
  Sum5 : Sum
  Out1 : Outport
  wires:
  In1/1 -> Gain5/1, Gain4/1
  Sum5/1 -> Out1/1
  Sum4/1 -> Delay7/1
  Delay7/1 -> Sum5/2
  Gain4/1 -> Sum5/1, Delay6/1
  Gain5/1 -> Sum4/1
  Delay6/1 -> Sum4/2

== system MIMO_FLOATING_POINT/Transceiver7/Interpolation 1/E7 ==
  In1 : Inport
  Delay6 : Delay  DelayLength=1
  Delay7 : Delay  DelayLength=1
  Gain4 : Gain  Gain=56
  Gain5 : Gain  Gain=336
  Gain6 : Gain  Gain=120
  Sum4 : Sum
  Sum5 : Sum
  Out1 : Outport
  wires:
  Gain4/1 -> Delay6/1
  In1/1 -> Gain6/1, Gain5/1, Gain4/1
  Sum5/1 -> Out1/1
  Sum4/1 -> Delay7/1
  Delay7/1 -> Sum5/2
  Gain6/1 -> Sum5/1
  Gain5/1 -> Sum4/1
  Delay6/1 -> Sum4/2
